simulink model "Tank_System"  (R2013b)
settings: Solver=ode45  StartTime=0.0  StopTime=10.0  RelTol=1e-3
settings Model: Creator=MMSA  LastModifiedBy=MMSA
settings SolverCC: ZeroCrossAlgorithm=Adaptive  PositivePriorityOrder=on
settings HardwareCC: ProdBitPerPointer=64  ProdHWDeviceType=Generic->64-bit Embedded Processor (LLP64)

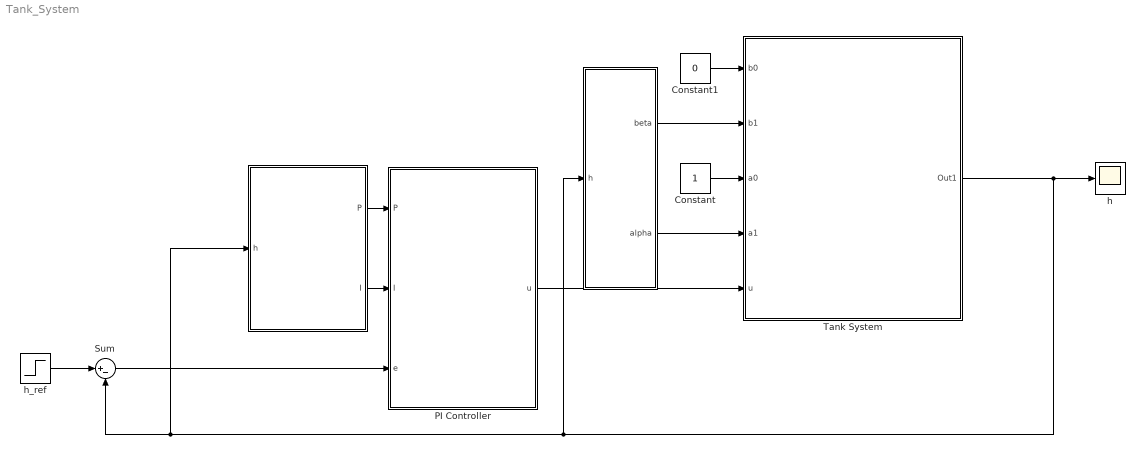
== system Tank_System ==
  " " : MATLAB Function  TreatAsAtomicUnit=on
  "  " : MATLAB Function  TreatAsAtomicUnit=on
  Constant : Constant
  Constant1 : Constant  Value=0
  PI Controller : Subsystem
  Sum : Sum  Inputs=|+-
  Tank System : Subsystem
  h : Scope
  h_ref : Step  Time=5  Before=10  After=20  SampleTime=0
  wires:
  PI Controller/1(u) -> Tank System/5(u)
  Sum/1 -> PI Controller/3(e)
  h_ref/1 -> Sum/1
  Tank System/1(Out1) -> " "/1(h), "  "/1(h), Sum/2, h/1
  Constant/1 -> Tank System/3(a0)
  Constant1/1 -> Tank System/1(b0)
  " "/2(alpha) -> Tank System/4(a1)
  " "/1(beta) -> Tank System/2(b1)
  "  "/1(P) -> PI Controller/1(P)
  "  "/2(I) -> PI Controller/2(I)

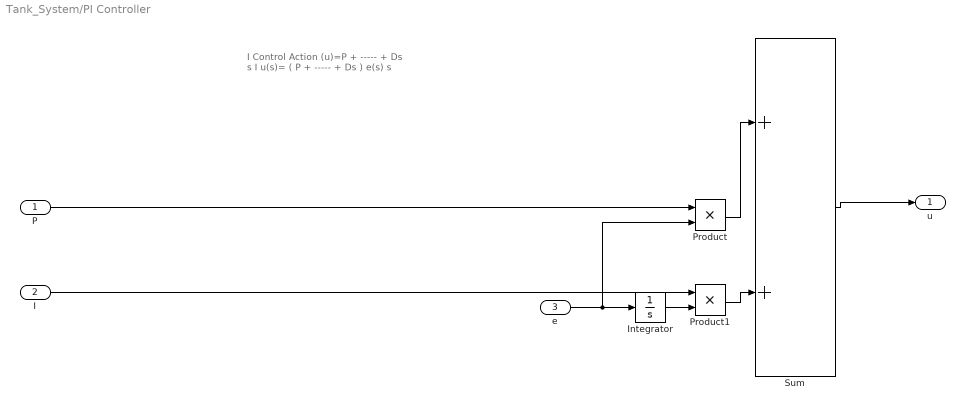
== system Tank_System/PI Controller ==
  note: I
      | Control Action (u)=P +  ----- + Ds
      |                                         s
      |                        I
      |    u(s)= ( P + ----- + Ds ) e(s)
      |                        s
  P : Inport
  I : Inport  Port=2
  e : Inport  Port=3
  Integrator : Integrator
  Product : Product
  Product1 : Product
  Sum : Sum  Inputs=|++
  u : Outport
  wires:
  I/1 -> Product1/1
  P/1 -> Product/1
  Sum/1 -> u/1
  Product/1 -> Sum/1
  e/1 -> Product/2, Integrator/1
  Integrator/1 -> Product1/2
  Product1/1 -> Sum/2

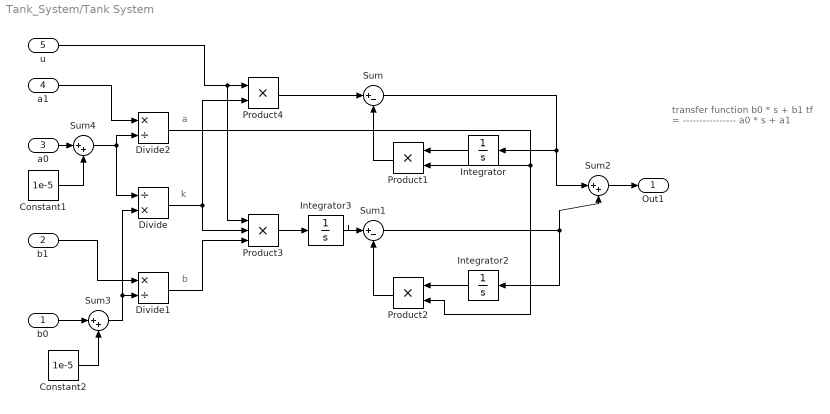
== system Tank_System/Tank System ==
  note: transfer function
      |       b0 * s + b1
      | tf = ----------------
      |       a0 * s + a1
  note: b
  note: a
  note: k
  b0 : Inport
  b1 : Inport  Port=2
  a0 : Inport  Port=3
  a1 : Inport  Port=4
  u : Inport  Port=5
  Constant1 : Constant  Value=1e-5
  Constant2 : Constant  Value=1e-5
  Divide : Product  Inputs=/*
  Divide1 : Product  Inputs=*/
  Divide2 : Product  Inputs=*/
  Integrator : Integrator
  Integrator2 : Integrator
  Integrator3 : Integrator
  Product1 : Product
  Product2 : Product
  Product3 : Product  Inputs=3
  Product4 : Product
  Sum : Sum  Inputs=|+-
  Sum1 : Sum  Inputs=|+-
  Sum2 : Sum  Inputs=|++
  Sum3 : Sum  Inputs=|++
  Sum4 : Sum  Inputs=|++
  Out1 : Outport
  wires:
  Integrator/1 -> Product1/1
  Product1/1 -> Sum/2
  Sum/1 -> Sum2/1, Integrator/1
  Product4/1 -> Sum/1
  b1/1 -> Divide1/1
  a1/1 -> Divide2/1
  Divide2/1 -> Product2/2, Product1/2
  Divide1/1 -> Product3/3
  Integrator2/1 -> Product2/1
  Product2/1 -> Sum1/2
  Sum1/1 -> Sum2/2, Integrator2/1
  Integrator3/1 -> Sum1/1
  Product3/1 -> Integrator3/1
  Divide/1 -> Product4/2, Product3/2
  u/1 -> Product4/1, Product3/1
  Sum2/1 -> Out1/1
  Constant2/1 -> Sum3/2
  b0/1 -> Sum3/1
  Sum3/1 -> Divide/2, Divide1/2
  a0/1 -> Sum4/1
  Sum4/1 -> Divide2/2, Divide/1
  Constant1/1 -> Sum4/2

== matlab function Tank_System/  ==
  data: h input; beta output; alpha output
function [beta, alpha] = TankTF(h)
%{
 this function is used to comute the tank transfer function parameter
                   beta
G(s) = ----------------
              s  +  alpha
%}
%% Coded by
% Mohamed Mohamed El-Sayed Atyya
% mohamed.atyya94@eng-st.cu.edu.eg
%% function body
% A(0)
A0=20;
% tap cross sectional area
a=2;
% gravity
g=9.81;
if h == 0
    h=1e-5;
end
% Area with different  h as the area law : A(h) = A(0) + h^2
Ah=A0+h^2;
% TF parameter
beta=1/Ah;
alpha=a/2/Ah*sqrt(2*g/abs(h));
end

== matlab function Tank_System/   ==
  data: h input; P output; I output
function [P, I] = PI(h)
%{
      this function is used to comute the controller parameter 
                               I       
       Gc(s) = P + ------
                              s
%}
%% Coded by
% Mohamed Mohamed El-Sayed Atyya
% mohamed.atyya94@eng-st.cu.edu.eg
%% function body
% A(0) must be equal with the other in TankTF function
A0=20;
% closed characteristics
zeta=0.7;
wn=4;
% Area with different  h as the area law : A(h) = A(0) + h^2  must be equal with the other in TankTF function
Ah=A0+h^2;
% Controller parameter
P=2*zeta*wn*Ah;
Ti=2*zeta/wn;
I=P/Ti;
end
